simulink model "main_STM32_H743_MIL"  (R2023b)
settings: Solver=VariableStepAuto  StartTime=0.0  StopTime=6  MaxStep=1e-1  RelTol=1e-3  EnableMultiTasking=on
undefined symbols (not defined in the file): b_vkm, c1_vsens, c3_vsens, DiscIntNeverNeededParam, iG_car, k1, k2, k3, k4, k5, m_vkm, p, v_0
libraries: simulink x5
settings Model: Creator=Sascha  LastModifiedBy=Sascha
settings SolverCC: ZeroCrossAlgorithm=Adaptive  AlgebraicLoopSolver=TrustRegion
settings OptimizationCC: DefaultParameterBehavior=Inlined  EnhancedBackFolding=on  PassReuseOutputArgsAs=Individual arguments  ZeroExternalMemoryAtStartup=off  ZeroInternalMemoryAtStartup=off  MaxStackSize=64  OptimizeBlockOrder=speed  DifferentSizesBufferReuse=on  OptimizationCustomize=off  EfficientTunableParamExpr=on
settings DebuggingCC: IgnoredZcDiagnostic=none  ParameterTunabilityLossMsg=error  UnconnectedInputMsg=warning  UnconnectedOutputMsg=warning  UnconnectedLineMsg=warning
settings HardwareCC: ProdBitPerPointer=32  ProdBitPerSizeT=32  ProdBitPerPtrDiffT=32  ProdLargestAtomicInteger=Long  ProdLargestAtomicFloat=Double  ProdWordSize=32  ProdLongLongMode=on  ProdHWDeviceType=ARM Compatible->ARM Cortex
settings ModelReferenceCC: EnableRefExpFcnMdlSchedulingChecks=on
settings SFSimCC: MATLABDynamicMemAlloc=off
settings RTWCC: Description=Embedded Coder  SystemTargetFile=ert.tlc  TemplateMakefile=ert_default_tmf  Toolchain=GNU Tools for ARM Embedded Processors  DLArmComputeVersion=19.05
settings CodeAppCC: ForceParamTrailComments=on  IgnoreCustomStorageClasses=off  OperatorAnnotations=on  SimulinkDataObjDesc=on  SFDataObjDesc=on  InsertBlockDesc=on
settings ERTTargetCC: ExtModeTransport=3  ExtModeStaticAlloc=on  ExtModeStaticAllocSize=5000  ExtModeMexFile=ext_xcp  ExtModeIntrfLevel=Level2 - Open  InlinedParameterPlacement=NonHierarchical  ERTCustomFileTemplate=example_file_process.tlc

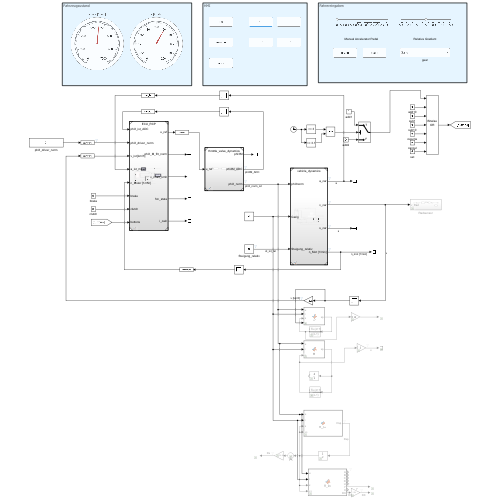
[thumbnail: Simulink's stored preview of the top-level diagram]
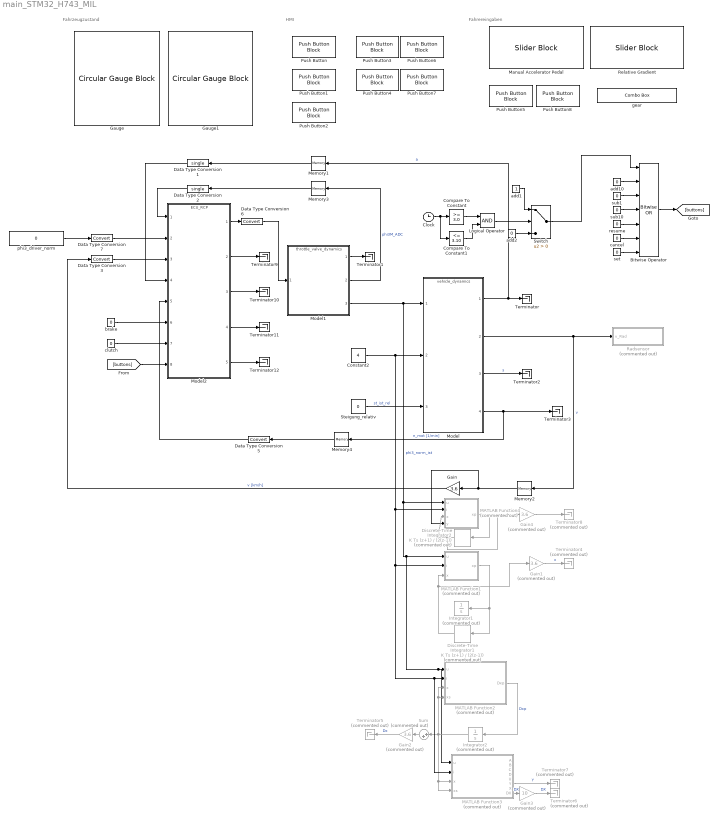
== system main_STM32_H743_MIL ==
  note: HMI
  note: Fahrzeugzustand
  note: Fahrereingaben
  Bitwise Operator : simulink/Logic and Bit Operations/Bitwise Operator  logicop=OR  UseBitMask=off  NumInputPorts=7  BitMask=bin2dec('11011001')  BitMaskRealWorld=Stored Integer
  Clock : Clock
  Compare To Constant : simulink/Logic and Bit Operations/Compare To Constant  relop=>=  const=3.0  OutDataTypeStr=boolean
  Compare To Constant1 : simulink/Logic and Bit Operations/Compare To Constant  relop=<=  const=3.10  OutDataTypeStr=boolean
  Constant2 : Constant  Value=4
  Data Type Conversion1 : DataTypeConversion  OutDataTypeStr=single  SaturateOnIntegerOverflow=off  RndMeth=Floor
  Data Type Conversion2 : DataTypeConversion  OutDataTypeStr=single  SaturateOnIntegerOverflow=off  RndMeth=Floor
  Data Type Conversion{3,5..7} (4 alike) : DataTypeConversion  SaturateOnIntegerOverflow=off  RndMeth=Floor
  Discrete-Time Integrator1 : DiscreteIntegrator  Commented=on  IntegratorMethod=Integration: Trapezoidal  InitialCondition=v_0  SampleTime=0.1  ICPrevOutput=DiscIntNeverNeededParam  ICPrevScaledInput=DiscIntNeverNeededParam
  Discrete-Time Integrator2 : DiscreteIntegrator  Commented=on  IntegratorMethod=Integration: Trapezoidal  InitialCondition=v_0  SampleTime=0.1  ICPrevOutput=DiscIntNeverNeededParam  ICPrevScaledInput=DiscIntNeverNeededParam
  Gain : Gain  Gain=3.6
  Gain1 : Gain  Commented=on  Gain=3.6
  Gain2 : Gain  Commented=on  Gain=3.6
  Gain3 : Gain  Commented=on  Gain=10
  Gain4 : Gain  Commented=on  Gain=3.6
  Gauge : CircularGaugeBlock  ScaleMax=7000  TickInterval=1000
  Gauge1 : CircularGaugeBlock  ScaleMax=200  TickInterval=20
  Integrator1 : Integrator  Commented=on  InitialCondition=v_0
  Integrator2 : Integrator  Commented=on  InitialCondition=v_0
  Logical Operator : Logic  AllPortsSameDT=off  OutDataTypeStr=boolean
  MATLAB Function1 : MATLAB Function  Commented=on  TreatAsAtomicUnit=on
  MATLAB Function2 : MATLAB Function  Commented=on  TreatAsAtomicUnit=on
  MATLAB Function3 : MATLAB Function  Commented=on  TreatAsAtomicUnit=on
  MATLAB Function4 : MATLAB Function  Commented=on  TreatAsAtomicUnit=on
  Manual Accelerator Pedal : SliderBlock  LabelPosition=Hide  ScaleMax=1
  Memory1 : Memory
  Memory2 : Memory  InitialCondition=v_0
  Memory3 : Memory
  Memory4 : Memory
  Model : ModelReference  ModelNameDialog=vehicle_dynamics.slx  SimulationMode=Normal  ModelReferenceVersion=7.0
  Model1 : ModelReference  ModelNameDialog=throttle_valve_dynamics.slx  SimulationMode=Normal  ModelReferenceVersion=6.0
  Model2 : ModelReference  ModelNameDialog=ECU_RCP.slx  SimulationMode=Normal  ModelReferenceVersion=7.19
  Push Button : PushButtonBlock  ButtonText=set  OffValue=0.000000
  Push Button1 : PushButtonBlock  ButtonText=resume  OnValue=5  OffValue=0.000000
  Push Button2 : PushButtonBlock  ButtonText=cancel  OnValue=6  OffValue=0.000000
  Push Button3 : PushButtonBlock  ButtonText=+ 1  OffValue=0.000000
  Push Button4 : PushButtonBlock  ButtonText=+10  OnValue=2  OffValue=0.000000
  Push Button5 : PushButtonBlock  ButtonText=clutch  OffValue=0.000000
  Push Button6 : PushButtonBlock  ButtonText=- 1  OnValue=3  OffValue=0.000000
  Push Button7 : PushButtonBlock  ButtonText=- 10  OnValue=4  OffValue=0.000000
  Push Button8 : PushButtonBlock  ButtonText=brake  OffValue=0.000000
  Radsensor : Subsystem  Commented=on
  Relative Gradient : SliderBlock  LabelPosition=Hide  ScaleMin=-0.3  ScaleMax=0.3
  Steigung_relativ : Constant  Value=0
  Sum : Sum  Commented=on  Inputs=|++
  Switch : Switch  Criteria=u2 > Threshold  SaturateOnIntegerOverflow=off  InputSameDT=off
  Terminator{,1..3,9..12} (8 alike) : Terminator
  Terminator{4..8} (5 alike) : Terminator  Commented=on
  add1 : Constant  OutDataTypeStr=uint8
  add10 : Constant  Value=0  OutDataTypeStr=uint8
  add2 : Constant  Value=0  OutDataTypeStr=uint8
  brake : Constant  Value=0  OutDataTypeStr=uint8
  cancel : Constant  Value=0  OutDataTypeStr=uint8
  clutch : Constant  Value=0  OutDataTypeStr=uint8
  gear : ComboBox  LabelPosition=Hide  SelectedLabel=Gang 4
      settings: Values={{'Approx. Leerlauf', 'Gang 1', 'Gang 2', 'Gang 3', 'Gang 4', 'Gang 5'}, [0 1 2 3 4 5]}
  phi3_driver_norm : Constant  Value=0
  resume : Constant  Value=0  OutDataTypeStr=uint8
  set : Constant  Value=0  OutDataTypeStr=uint8
  sub1 : Constant  Value=0  OutDataTypeStr=uint8
  sub10 : Constant  Value=0  OutDataTypeStr=uint8
  wires:
  Model/1 -> Terminator/1, Memory1/1  "a"
  Model/2 -> Memory2/1, Radsensor/1(v_Rad)  "v"
  Model/3 -> Terminator2/1  "s"
  Model/4 -> Terminator3/1, Memory4/1  "n_mot [1/min]"
  Gain/1 -> Data Type Conversion3/1  "v [km/h]"
  Model2/1 -> Data Type Conversion6/1
  Model1/2 -> Memory3/1  "phi3M_ADC"
  Model1/3 -> MATLAB Function3/1(u), MATLAB Function2/1(u), MATLAB Function1/1(u), MATLAB Function4/1(u), Model/1  "phi3_norm_ist"
  Model1/1 -> Terminator1/1
  Memory2/1 -> MATLAB Function4/4(y), Gain/1
  Memory3/1 -> Data Type Conversion2/1
  Memory4/1 -> Data Type Conversion5/1
  Switch/1 -> Bitwise Operator/1
  add10/1 -> Bitwise Operator/2
  sub1/1 -> Bitwise Operator/3
  sub10/1 -> Bitwise Operator/4
  Bitwise Operator/1 -> [buttons]
  [buttons] -> Model2/8
  clutch/1 -> Model2/7
  brake/1 -> Model2/6
  Data Type Conversion3/1 -> Model2/3
  Data Type Conversion5/1 -> Model2/5
  Data Type Conversion6/1 -> Model1/1
  phi3_driver_norm/1 -> Data Type Conversion7/1
  Data Type Conversion7/1 -> Model2/2
  Gain1/1 -> Terminator4/1  "x"
  MATLAB Function1/1(xp) -> Discrete-Time Integrator1/1, Integrator1/1
  Discrete-Time Integrator1/1 -> Gain1/1, MATLAB Function1/3(x)
  MATLAB Function2/1(Dxp) -> Integrator2/1  "Dxp"
  Integrator2/1 -> MATLAB Function2/4(xs), MATLAB Function2/3(x), MATLAB Function3/3(x), MATLAB Function3/4(xs), Sum/1
  Constant2/1 -> MATLAB Function3/2(i), MATLAB Function2/2(i), MATLAB Function1/2(i), MATLAB Function4/2(i), Model/2
  Gain2/1 -> Terminator5/1  "Dx"
  Sum/1 -> Gain2/1
  Data Type Conversion1/1 -> Model2/4
  Memory1/1 -> Data Type Conversion1/1
  Gain3/1 -> Terminator6/1  "DX"
  MATLAB Function3/6(Y) -> Terminator7/1  "Y"
  MATLAB Function3/8(DX) -> Gain3/1  "DX"
  Steigung_relativ/1 -> Model/3  "st_ist_rel"
  Discrete-Time Integrator2/1 -> Gain4/1, MATLAB Function4/3(x)
  MATLAB Function4/1(xp) -> Discrete-Time Integrator2/1
  Gain4/1 -> Terminator8/1
  resume/1 -> Bitwise Operator/5
  cancel/1 -> Bitwise Operator/6
  set/1 -> Bitwise Operator/7
  Model2/2 -> Terminator9/1
  Model2/3 -> Terminator10/1
  Model2/4 -> Terminator11/1
  Model2/5 -> Terminator12/1
  Data Type Conversion2/1 -> Model2/1
  Clock/1 -> Compare To Constant1/1, Compare To Constant/1
  Compare To Constant/1 -> Logical Operator/1
  Compare To Constant1/1 -> Logical Operator/2
  Logical Operator/1 -> Switch/2
  add1/1 -> Switch/1
  add2/1 -> Switch/3

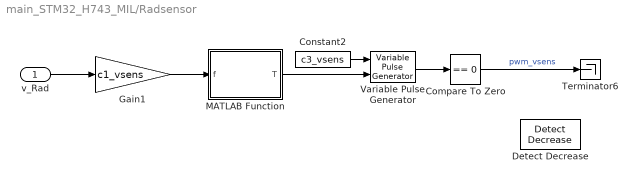
== system main_STM32_H743_MIL/Radsensor ==
  v_Rad : Inport
  Compare To Zero : simulink/Logic and Bit Operations/Compare To Zero  relop===  OutDataTypeStr=boolean
  Constant2 : Constant  Value=c3_vsens
  Detect Decrease : simulink/Logic and Bit Operations/Detect Decrease  vinit=0.0  OutDataTypeStr=boolean
  Gain1 : Gain  Gain=c1_vsens
  MATLAB Function : MATLAB Function  TreatAsAtomicUnit=on
  Terminator6 : Terminator
  Variable Pulse Generator : VariablePulseGenerator  AllowZeroPulseWidth=on  SampleTime=0.1
  wires:
  MATLAB Function/1(T) -> Variable Pulse Generator/2
  Constant2/1 -> Variable Pulse Generator/1
  Gain1/1 -> MATLAB Function/1(f)
  v_Rad/1 -> Gain1/1
  Variable Pulse Generator/1 -> Compare To Zero/1
  Compare To Zero/1 -> Terminator6/1  "pwm_vsens"

== matlab function main_STM32_H743_MIL/MATLAB Function3 ==
  data: A output; k1 parameter; k2 parameter; k3 parameter; k4 parameter; k5 parameter; u input; i input; p parameter; m_vkm parameter; b_vkm parameter; x input; iG_car parameter; xs input; B output; C output; D output; U output; Y output; X output; DX output
function [A,B,C,D,U,Y,X,DX] = ff_lin(k1, k2, k3, k4, k5, u, i, p, m_vkm, b_vkm, x, iG_car, xs)

% xs = 130/3.6;
% i = 4;

Ts = 0.1;

us = ((k1*xs^2+k2*xs+k3)*1/(k4*iG_car(i+1))-m_vkm*k5*iG_car(i+1)*xs-b_vkm)*1/(p(1)*k5^2*iG_car(i+1)^2*xs^2+p(2)*k5*iG_car(i+1)*xs+p(3));

Ac = [(-2*k1*xs-k2+2*k4*iG_car(i+1)^3*p(1)*k5^2*xs*us+k4*iG_car(i+1)^2*p(2)*k5*us+k4*iG_car(i+1)^2*m_vkm*k5)];
Bc = [(k4*iG_car(i+1)^3*p(1)*k5^2*xs^2+k4*iG_car(i+1)^2*p(2)*k5*xs+k4*iG_car(i+1)*p(3))];
Cc = [1];
Dc = [0];

nx = 1;
nu = 1;

M = expm([[Ac Bc]*Ts; zeros(nu,nx+nu)]);
A = M(1:nx,1:nx);
B = M(1:nx,nx+1:nx+nu);
C = Cc;
D = Dc;

X = x;
U = u;
Y = C*x+D*u;
DX = A*x+B*u-x;

% DX = (-2*k1*xs-k2+2*k4*iG_car(i+1)^3*p(1)*k5^2*xs*us+k4*iG_car(i+1)^2*p(2)*k5*us+k4*iG_car(i+1)^2*m_vkm*k5) * (x-xs)  +   (k4*iG_car(i+1)^3*p(1)*k5^2*xs^2+k4*iG_car(i+1)^2*p(2)*k5*xs+k4*iG_car(i+1)*p(3)) * (u-us);

== matlab function main_STM32_H743_MIL/Radsensor/MATLAB Function ==
  data: f input; T output
function T = freq2time(f)
    if f > 0
        T = 1/f;
    else
        T = 0;
    end

== matlab function main_STM32_H743_MIL/MATLAB Function1 ==
  data: xp output; k1 parameter; k2 parameter; k3 parameter; k4 parameter; k5 parameter; u input; i input; p parameter; m_vkm parameter; b_vkm parameter; x input; iG_car parameter
function xp = ff(k1, k2, k3, k4, k5, u, i, p, m_vkm, b_vkm, x, iG_car)

xp = -k1*x^2-k2*x-k3+k4*iG_car(i+1)*((p(1)*k5^2*iG_car(i+1)^2*x^2+p(2)*k5*iG_car(i+1)*x+p(3))*u+m_vkm*k5*iG_car(i+1)*x+b_vkm);

== matlab function main_STM32_H743_MIL/MATLAB Function2 ==
  data: Dxp output; k1 parameter; k2 parameter; k3 parameter; k4 parameter; k5 parameter; u input; i input; p parameter; m_vkm parameter; b_vkm parameter; x input; iG_car parameter; xs input
function Dxp = ff_lin(k1, k2, k3, k4, k5, u, i, p, m_vkm, b_vkm, x, iG_car, xs)

% xs = 130/3.6;

us = ((k1*xs^2+k2*xs+k3)*1/(k4*iG_car(i+1))-m_vkm*k5*iG_car(i+1)*xs-b_vkm)*1/(p(1)*k5^2*iG_car(i+1)^2*xs^2+p(2)*k5*iG_car(i+1)*xs+p(3));

Dxp = (-2*k1*xs-k2+2*k4*iG_car(i+1)^3*p(1)*k5^2*xs*us+k4*iG_car(i+1)^2*p(2)*k5*us+k4*iG_car(i+1)^2*m_vkm*k5) * (x-xs)  +   (k4*iG_car(i+1)^3*p(1)*k5^2*xs^2+k4*iG_car(i+1)^2*p(2)*k5*xs+k4*iG_car(i+1)*p(3)) * (u-us);

== matlab function main_STM32_H743_MIL/MATLAB Function4 ==
  data: xp output; k1 parameter; k2 parameter; k3 parameter; k4 parameter; k5 parameter; u input; i input; p parameter; m_vkm parameter; b_vkm parameter; x input; iG_car parameter; y input
function xp = ff(k1, k2, k3, k4, k5, u, i, p, m_vkm, b_vkm, x, iG_car, y)

k = 1;
y_hat = x;

xp = -k1*x^2-k2*x-k3+k4*iG_car(i+1)*((p(1)*k5^2*iG_car(i+1)^2*x^2+p(2)*k5*iG_car(i+1)*x+p(3))*u+m_vkm*k5*iG_car(i+1)*x+b_vkm)   + k*(y-y_hat);
